simulink model "DSXH111"  (R2018b)
settings: Solver=VariableStepAuto  StartTime=0.0  StopTime=10  RelTol=1e-3
undefined symbols (not defined in the file): magnitude
libraries: simulink x1
settings Model: Creator=ASUS  LastModifiedBy=DELL
settings DataIOCC: ReturnWorkspaceOutputs=on
settings DebuggingCC: UnconnectedInputMsg=none  UnconnectedOutputMsg=none  UnconnectedLineMsg=none

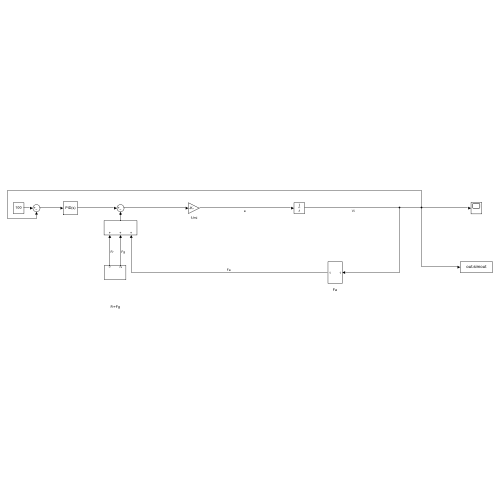
[thumbnail: Simulink's stored preview of the top-level diagram]
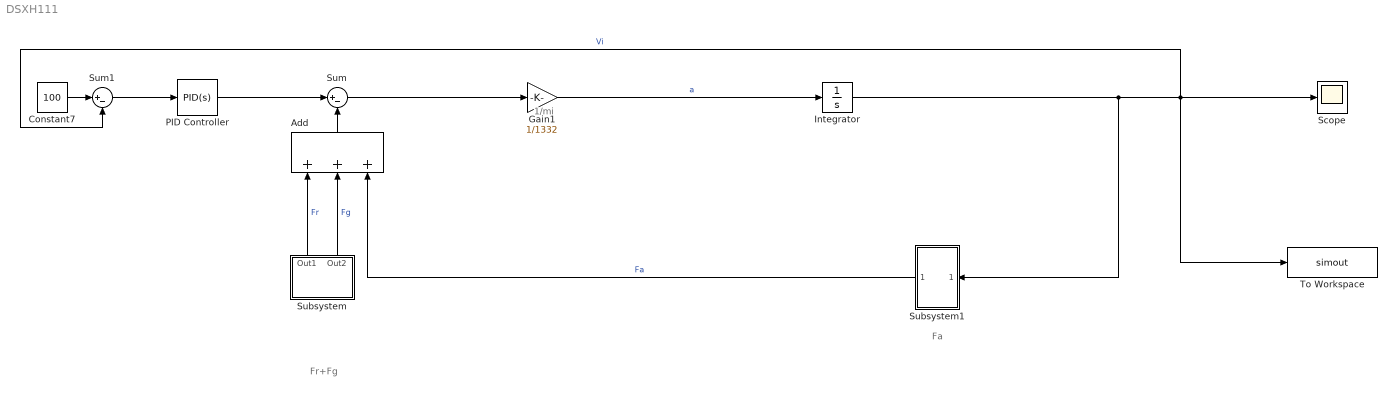
== system DSXH111 ==
  note: Fa
  note: Fr+Fg
  note: 1/mi
  Add : Sum  Inputs=3
  Constant7 : Constant  Value=100
  Gain1 : Gain  Gain=1/1332
  Integrator : Integrator
  PID Controller : simulink/Continuous/PID Controller  Controller=PID  Form=Parallel  TimeDomain=Continuous-time  SampleTime=-1  IntegratorMethod=Forward Euler  ControllerParametersSource=internal  P=3195.5082683321  I=1423.88479583913  D=-84.9618302848476  N=4.12705470337619  UseFilter=on  TunerSelectOption=Transfer Function Based (PID Tuner App)  InitialConditionSource=internal  InitialConditionForIntegrator=0  InitialConditionForFilter=0  DifferentiatorICPrevScaledInput=0  ExternalReset=none  TrackingMode=off  Kt=1  LimitOutput=off  UpperSaturationLimit=inf  LowerSaturationLimit=-inf  LinearizeAsGain=on  AntiWindupMode=none  Kb=1  POutMin=[]  POutMax=[]  IOutMin=[]  IOutMax=[]  DOutMin=[]  DOutMax=[]  NOutMin=[]  NOutMax=[]  SumOutMin=[]  SumOutMax=[]  SaturationOutMin=[]  SaturationOutMax=[]  PParamMin=[]  PParamMax=[]  IParamMin=[]  IParamMax=[]  DParamMin=[]  DParamMax=[]  NParamMin=[]  NParamMax=[]  KbParamMin=[]  KbParamMax=[]  KtParamMin=[]  KtParamMax=[]  KbOutMin=[]  KbOutMax=[]  KtOutMin=[]  KtOutMax=[]  IntegratorOutMin=[]  IntegratorOutMax=[]  FilterOutMin=[]  FilterOutMax=[]  SumI1OutMin=[]  SumI1OutMax=[]  SumI2OutMin=[]  SumI2OutMax=[]  SumI3OutMin=[]  SumI3OutMax=[]  SumI4OutMin=[]  SumI4OutMax=[]  SumDOutMin=[]  SumDOutMax=[]  DifferentiatorOutMin=[]  DifferentiatorOutMax=[]  FilterDiffOutCoefMin=[]  FilterDiffOutCoefMax=[]  ReciprocalOutMin=[]  ReciprocalOutMax=[]  SumDenOutMin=[]  SumDenOutMax=[]  SumNumOutMin=[]  SumNumOutMax=[]  DivideOutMin=[]  DivideOutMax=[]  IntegratorContinuousStateAttributes=''  IntegratorStateMustResolveToSignalObject=off  IntegratorRTWStateStorageClass=Auto  FilterContinuousStateAttributes=''  FilterStateMustResolveToSignalObject=off  FilterRTWStateStorageClass=Auto  ParallelPVariant=InternalParameters  IdealPVariant=Disabled  IVariant=InternalParameters  DVariant=InternalParameters  IntegratorVariant=Continuous  SatVariant=Disabled  AWVariant=Passthrough  PCopyVariant=Disabled  TRVariant=Disabled  FdbkBlocksVariant=Forward  IdealPFdbkVariant=Disabled  SatFdbkVariant=Disabled  DerivativeFilterVariant=ContFilter  NVariant=InternalParameters  NCopyVariant=Disabled  FilterICVariant=InternalICsFilter  IntegratorICVariant=InternalICs  ExternalResetVariant=Disabled  TRSumVariant=Passthrough  SumFdbkVariant=Disabled  SumVariant=Sum_PID
  Scope : Scope
  Subsystem : Subsystem
  Subsystem1 : Subsystem
  Sum : Sum  Inputs=|+-
  Sum1 : Sum  Inputs=|+-
  To Workspace : ToWorkspace  VariableName=simout  SaveFormat=Timeseries  SampleTime=-1
  wires:
  Integrator/1 -> Subsystem1/1(In1), To Workspace/1, Scope/1, Sum1/2  "Vi"
  Gain1/1 -> Integrator/1  "a"
  Add/1 -> Sum/2
  Sum/1 -> Gain1/1
  Sum1/1 -> PID Controller/1
  Constant7/1 -> Sum1/1
  PID Controller/1 -> Sum/1
  Subsystem/1(Out1) -> Add/1  "Fr"
  Subsystem/2(Out2) -> Add/2  "Fg"
  Subsystem1/1(Out1) -> Add/3  "Fa"

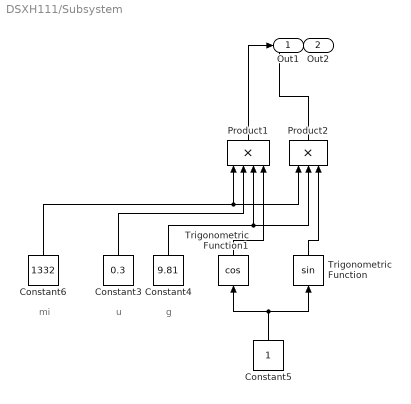
== system DSXH111/Subsystem ==
  note: mi
  note: g
  note: u
  Constant3 : Constant  Value=0.3
  Constant4 : Constant  Value=9.81
  Constant5 : Constant
  Constant6 : Constant  Value=1332
  Product1 : Product  Inputs=4
  Product2 : Product  Inputs=3
  Trigonometric Function : Trigonometry
  Trigonometric Function1 : Trigonometry  Operator=cos
  Out1 : Outport
  Out2 : Outport  Port=2
  wires:
  Constant5/1 -> Trigonometric Function/1, Trigonometric Function1/1
  Trigonometric Function1/1 -> Product1/4
  Constant6/1 -> Product2/1, Product1/1
  Product2/1 -> Out2/1
  Constant4/1 -> Product2/2, Product1/3
  Constant3/1 -> Product1/2
  Trigonometric Function/1 -> Product2/3
  Product1/1 -> Out1/1

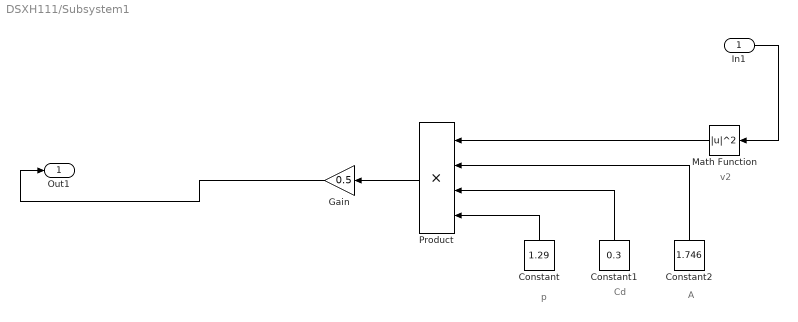
== system DSXH111/Subsystem1 ==
  note: p
  note: Cd
  note: A
  note: v2
  In1 : Inport
  Constant : Constant  Value=1.29
  Constant1 : Constant  Value=0.3
  Constant2 : Constant  Value=1.746
  Gain : Gain  Gain=0.5
  Math Function : Math  Operator=magnitude^2  SaturateOnIntegerOverflow=on
  Product : Product  Inputs=4
  Out1 : Outport
  wires:
  Constant2/1 -> Product/2
  Constant1/1 -> Product/3
  Gain/1 -> Out1/1
  Constant/1 -> Product/4
  In1/1 -> Math Function/1
  Product/1 -> Gain/1
  Math Function/1 -> Product/1
